simulink subsystem "reference_generator"  (R2020a)
settings: Solver=VariableStepAuto  StartTime=0.0  StopTime=10.0  RelTol=1e-3
model mask{x_params=0, y_params=0, depth_params=0, abs_yaw_params=0, distance=0, desired_lat_vel=0, lat_vel_error_gain=0, counter_max=0}
  mask prompts: x_params "X"; y_params "Y"; depth_params "Depth"; abs_yaw_params "Abs. Yaw"; distance "Distance from pylon"; desired_lat_vel "Desired Lat. Velocity"; lat_vel_error_gain "Lat. Velocity Error Gain"; counter_max "Number of transepts"
undefined symbols (not defined in the file): bool_inspection, misu_Ts, pylonCenter, speed
libraries: simulink x1
settings Model: Creator=andrea  LastModifiedBy=stefano

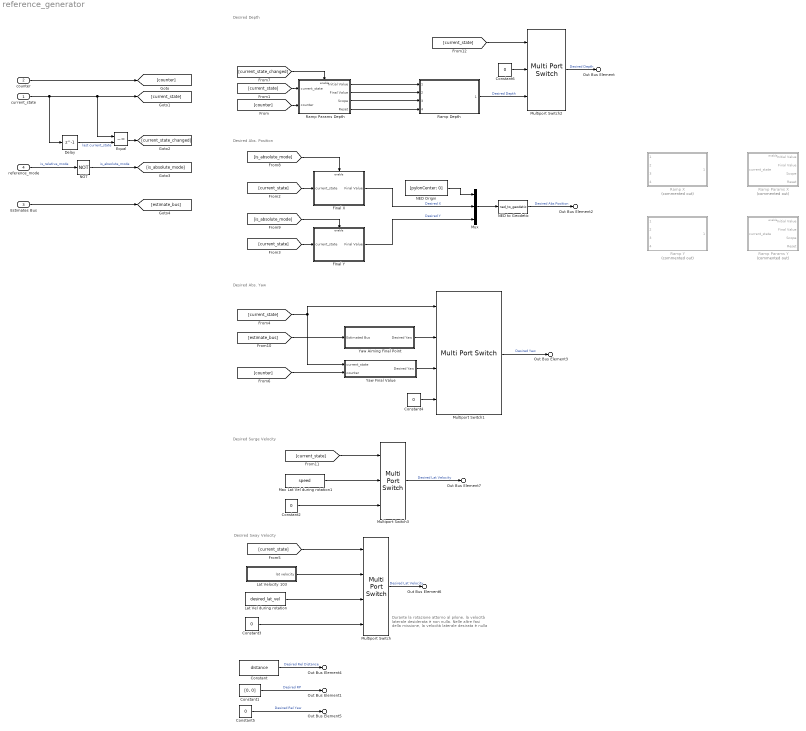
== system reference_generator ==
  note: Desired Surge Velocity
  note: Desired Abs. Yaw
  note: Desired Abs. Position
  note: Desired Depth
  note: Desired Sway Velocity
  note: Durante la rotazione attorno al pilone, la velocità laterale desiderata
      | è non nulla. Nelle altre fasi della missione, la velocità laterale desirata è nulla
  current_state : Inport
  counter : Inport  Port=2
  "Estimates Bus " : Inport  Port=3
  reference_mode : Inport  Port=4
  Constant : Constant  Value=distance
  Constant1 : Constant  Value=[0, 0]
  Constant{2..6} (5 alike) : Constant  Value=0
  Delay : Delay  DelayLength=1
  Equal : RelationalOperator  Operator=~=  OutDataTypeStr=boolean  RndMeth=Simplest
  FInal Y : Subsystem
  Final X : Subsystem
  Lat Vel during rotation : Constant  Value=desired_lat_vel
  Lat Velocity 103 : Subsystem
  Max Lat Vel during rotation1 : Constant  Value=speed
  Multiport Switch : MultiPortSwitch  DataPortOrder=Specify indices  DataPortIndices={103, 202, 201}  DiagnosticForDefault=None
  Multiport Switch1 : MultiPortSwitch  DataPortOrder=Specify indices  DataPortIndices={102, [101, 103, 104, 201, 202, 401]}  DataPortForDefault=Additional data port  DiagnosticForDefault=None
  Multiport Switch2 : MultiPortSwitch  DataPortOrder=Specify indices  DataPortIndices={500, 0}  DiagnosticForDefault=None
  Multiport Switch3 : MultiPortSwitch  DataPortOrder=Specify indices  DataPortIndices={[102], 201}  DiagnosticForDefault=None
  Mux : Mux  Inputs=3
  NED Origin : Constant  Value=[pylonCenter; 0]
  NED to Geodetic : MATLABFcn  MATLABFcn=ned_to_geodetic
  NOT : Logic  Operator=NOT  AllPortsSameDT=off  OutDataTypeStr=boolean
  Ramp Depth : Subsystem  ReferencedSubsystem=ramp_generator
  Ramp Params Depth : Subsystem
  Ramp Params X : Subsystem  Commented=on
  Ramp Params Y : Subsystem  Commented=on
  Ramp X : Subsystem  Commented=on  ReferencedSubsystem=ramp_generator
  Ramp Y : Subsystem  Commented=on  ReferencedSubsystem=ramp_generator
  Yaw Aiming Final Point : Subsystem
  Yaw Final Value : Subsystem
  Out Bus Element : Outport  PortName=Desired  Element=Depth
  Out Bus Element1 : Outport  PortName=Desired  Element=RollPitch
  Out Bus Element2 : Outport  PortName=Desired  Element=Abs Position
  Out Bus Element3 : Outport  PortName=Desired  Element=Yaw
  Out Bus Element4 : Outport  PortName=Desired  Element=Rel Distance
  Out Bus Element5 : Outport  PortName=Desired  Element=Rel Orientation
  Out Bus Element6 : Outport  PortName=Desired  Element=Sway Velocity
  Out Bus Element7 : Outport  PortName=Desired  Element=Surge Velocity
  wires:
  "Estimates Bus "/1 -> [estimate_bus]
  Ramp Params Depth/1(Initial Value) -> Ramp Depth/1
  Ramp Params Depth/4(Reset) -> Ramp Depth/4
  FInal Y/1(Final Value) -> Mux/3  "Desired Y"
  Constant/1 -> Out Bus Element4/1  "Desired Rel Distance"
  Constant5/1 -> Out Bus Element5/1  "Desired Rel Yaw"
  Final X/1(Final Value) -> Mux/2  "Desired X"
  Mux/1 -> NED to Geodetic/1
  Ramp Params Depth/3(Scope) -> Ramp Depth/3
  Ramp Depth/1 -> Multiport Switch2/3  "Desired Depth"
  Multiport Switch1/1 -> Out Bus Element3/1  "Desired Yaw"
  Constant1/1 -> Out Bus Element1/1  "Desired RP"
  Ramp Params Depth/2(Final Value) -> Ramp Depth/2
  current_state/1 -> Delay/1, [current_state], Equal/1
  counter/1 -> [counter]
  NED to Geodetic/1 -> Out Bus Element2/1  "Desired Abs Position"
  NED Origin/1 -> Mux/1
  [counter] -> Ramp Params Depth/2(counter)
  [current_state] -> Ramp Params Depth/1(current_state)
  [current_state] -> Final X/1(current_state)
  [current_state] -> FInal Y/1(current_state)
  [current_state] -> Multiport Switch1/1, Yaw Final Value/1(current_state)
  [counter] -> Yaw Final Value/2(counter)
  Delay/1 -> Equal/2  "last current_state"
  Equal/1 -> [current_state_changed]
  [current_state_changed] -> Ramp Params Depth/Enable
  reference_mode/1 -> NOT/1  "is_relative_mode"
  [is_absolute_mode] -> Final X/Enable
  NOT/1 -> [is_absolute_mode]  "is_absolute_mode"
  Multiport Switch/1 -> Out Bus Element6/1  "Desired Lat Velocity"
  [current_state] -> Multiport Switch/1
  Lat Vel during rotation/1 -> Multiport Switch/3
  Constant3/1 -> Multiport Switch/4
  Yaw Aiming Final Point/1(Desired Yaw) -> Multiport Switch1/2
  Yaw Final Value/1(Desired Yaw) -> Multiport Switch1/3
  Constant4/1 -> Multiport Switch1/4
  [estimate_bus] -> Yaw Aiming Final Point/1(Estimated Bus)
  [is_absolute_mode] -> FInal Y/Enable
  [current_state] -> Multiport Switch2/1
  Multiport Switch2/1 -> Out Bus Element/1  "Desired Depth"
  Constant6/1 -> Multiport Switch2/2
  Multiport Switch3/1 -> Out Bus Element7/1  "Desired Lat Velocity"
  Max Lat Vel during rotation1/1 -> Multiport Switch3/2
  Constant2/1 -> Multiport Switch3/3
  [current_state] -> Multiport Switch3/1
  Lat Velocity 103/1(lat velocity) -> Multiport Switch/2

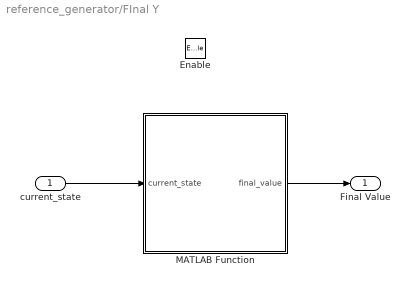
== system reference_generator/FInal Y ==
  current_state : Inport
  Enable : EnablePort
  MATLAB Function : MATLAB Function  TreatAsAtomicUnit=on
  Final Value : Outport
  wires:
  current_state/1 -> MATLAB Function/1(current_state)
  MATLAB Function/1(final_value) -> Final Value/1

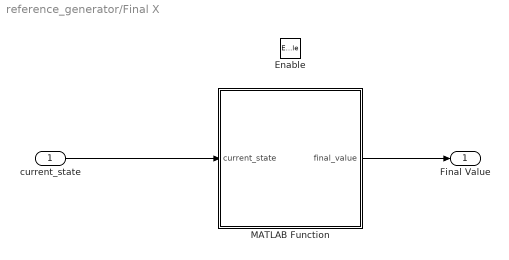
== system reference_generator/Final X ==
  current_state : Inport
  Enable : EnablePort
  MATLAB Function : MATLAB Function  TreatAsAtomicUnit=on
  Final Value : Outport
  wires:
  current_state/1 -> MATLAB Function/1(current_state)
  MATLAB Function/1(final_value) -> Final Value/1

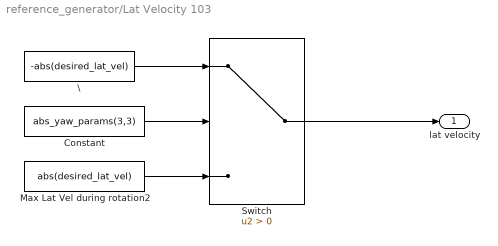
== system reference_generator/Lat Velocity 103 ==
  Constant : Constant  Value=abs_yaw_params(3,3)
  Max Lat Vel during rotation2 : Constant  Value=abs(desired_lat_vel)
  Switch : Switch  Criteria=u2 > Threshold
  \ : Constant  Value=-abs(desired_lat_vel)
  lat velocity : Outport
  wires:
  Switch/1 -> lat velocity/1
  \/1 -> Switch/1
  Max Lat Vel during rotation2/1 -> Switch/3
  Constant/1 -> Switch/2

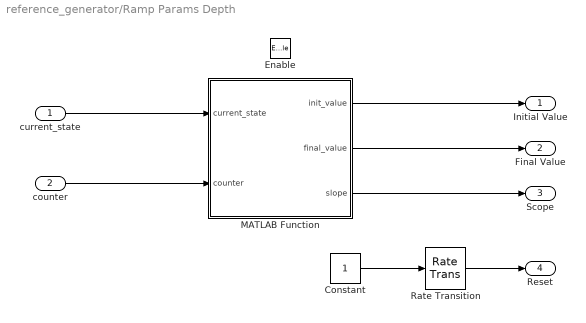
== system reference_generator/Ramp Params Depth ==
  current_state : Inport
  counter : Inport  Port=2
  Enable : EnablePort
  Constant : Constant
  MATLAB Function : MATLAB Function  TreatAsAtomicUnit=on
  Rate Transition : RateTransition  OutPortSampleTime=misu_Ts
  Initial Value : Outport
  Final Value : Outport  Port=2
  Scope : Outport  Port=3
  Reset : Outport  Port=4  OutputWhenDisabled=reset  InitialOutput=0
  wires:
  Rate Transition/1 -> Reset/1
  MATLAB Function/3(slope) -> Scope/1
  MATLAB Function/2(final_value) -> Final Value/1
  MATLAB Function/1(init_value) -> Initial Value/1
  Constant/1 -> Rate Transition/1
  counter/1 -> MATLAB Function/2(counter)
  current_state/1 -> MATLAB Function/1(current_state)

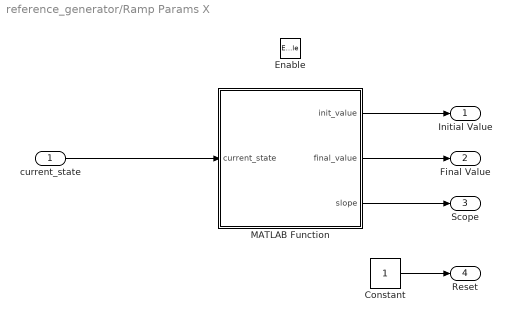
== system reference_generator/Ramp Params X ==
  current_state : Inport
  Enable : EnablePort
  Constant : Constant
  MATLAB Function : MATLAB Function  TreatAsAtomicUnit=on
  Initial Value : Outport
  Final Value : Outport  Port=2
  Scope : Outport  Port=3
  Reset : Outport  Port=4  OutputWhenDisabled=reset  InitialOutput=0
  wires:
  current_state/1 -> MATLAB Function/1(current_state)
  Constant/1 -> Reset/1
  MATLAB Function/3(slope) -> Scope/1
  MATLAB Function/2(final_value) -> Final Value/1
  MATLAB Function/1(init_value) -> Initial Value/1

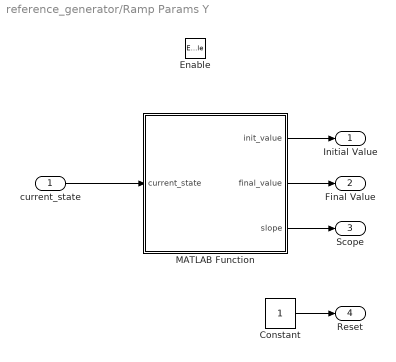
== system reference_generator/Ramp Params Y ==
  current_state : Inport
  Enable : EnablePort
  Constant : Constant
  MATLAB Function : MATLAB Function  TreatAsAtomicUnit=on
  Initial Value : Outport
  Final Value : Outport  Port=2
  Scope : Outport  Port=3
  Reset : Outport  Port=4  OutputWhenDisabled=reset  InitialOutput=0
  wires:
  current_state/1 -> MATLAB Function/1(current_state)
  Constant/1 -> Reset/1
  MATLAB Function/3(slope) -> Scope/1
  MATLAB Function/2(final_value) -> Final Value/1
  MATLAB Function/1(init_value) -> Initial Value/1

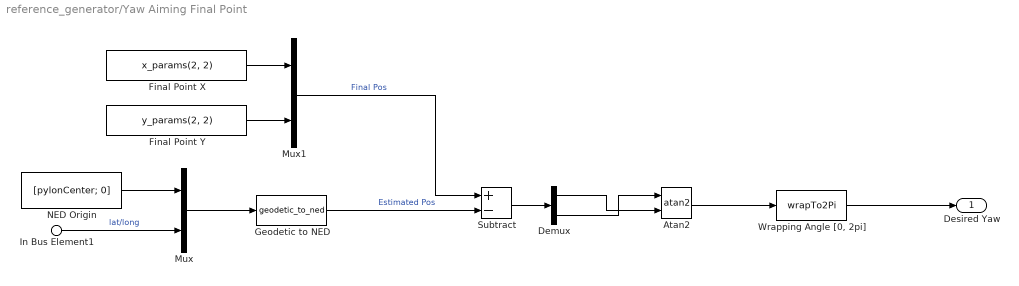
== system reference_generator/Yaw Aiming Final Point ==
  In Bus Element1 : Inport  PortName=Estimated Bus  Element=Estimated Abs Position
  Atan2 : Trigonometry  Operator=atan2
  Demux : Demux  Outputs=2
  Final Point X : Constant  Value=x_params(2, 2)
  Final Point Y : Constant  Value=y_params(2, 2)
  Geodetic to NED : MATLABFcn  MATLABFcn=geodetic_to_ned
  Mux : Mux  Inputs=2
  Mux1 : Mux  Inputs=2
  NED Origin : Constant  Value=[pylonCenter; 0]
  Subtract : Sum  Inputs=+-
  "Wrapping Angle [0, 2pi]" : MATLABFcn  MATLABFcn=wrapTo2Pi  OutputDimensions=1
  Desired Yaw : Outport
  wires:
  "Wrapping Angle [0, 2pi]"/1 -> Desired Yaw/1
  Atan2/1 -> "Wrapping Angle [0, 2pi]"/1
  Subtract/1 -> Demux/1
  Mux1/1 -> Subtract/1  "Final Pos"
  Final Point Y/1 -> Mux1/2
  Final Point X/1 -> Mux1/1
  Geodetic to NED/1 -> Subtract/2  "Estimated Pos"
  In Bus Element1/1 -> Mux/2  "lat/long"
  Mux/1 -> Geodetic to NED/1
  NED Origin/1 -> Mux/1
  Demux/1 -> Atan2/2
  Demux/2 -> Atan2/1

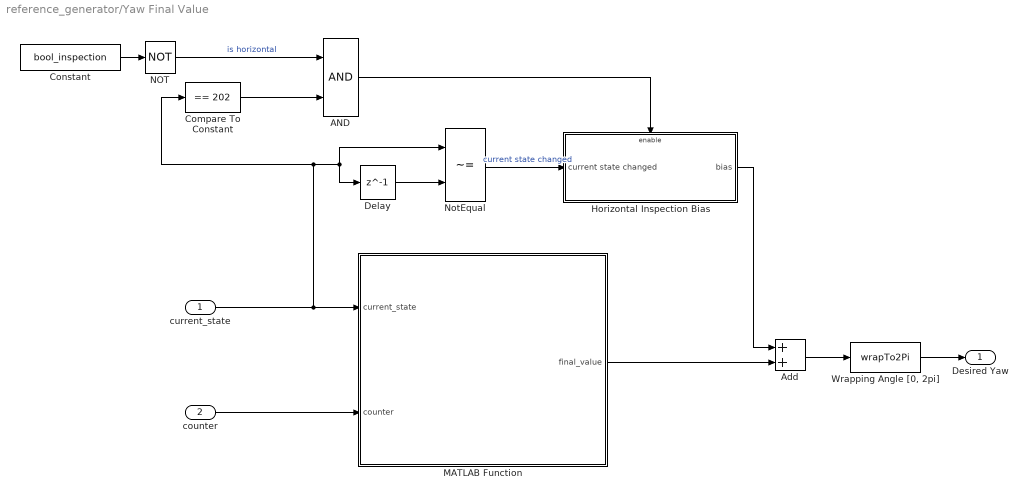
== system reference_generator/Yaw Final Value ==
  current_state : Inport
  counter : Inport  Port=2
  AND : Logic  IconShape=distinctive  AllPortsSameDT=off  OutDataTypeStr=boolean
  Add : Sum
  Compare To Constant : simulink/Logic and Bit Operations/Compare To Constant  relop===  const=202  OutDataTypeStr=boolean
  Constant : Constant  Value=bool_inspection
  Delay : Delay  DelayLength=1
  Horizontal Inspection Bias : Subsystem
  MATLAB Function : MATLAB Function  TreatAsAtomicUnit=on
  NOT : Logic  Operator=NOT  IconShape=distinctive  AllPortsSameDT=off  OutDataTypeStr=boolean
  NotEqual : RelationalOperator  Operator=~=  OutDataTypeStr=boolean  RndMeth=Simplest
  "Wrapping Angle [0, 2pi]" : MATLABFcn  MATLABFcn=wrapTo2Pi
  Desired Yaw : Outport
  wires:
  NotEqual/1 -> Horizontal Inspection Bias/1(current state changed)  "current state changed"
  Delay/1 -> NotEqual/2
  current_state/1 -> MATLAB Function/1(current_state), Delay/1, NotEqual/1, Compare To Constant/1
  AND/1 -> Horizontal Inspection Bias/Enable
  Compare To Constant/1 -> AND/2
  NOT/1 -> AND/1  "is horizontal"
  Constant/1 -> NOT/1
  Horizontal Inspection Bias/1(bias) -> Add/1
  "Wrapping Angle [0, 2pi]"/1 -> Desired Yaw/1
  Add/1 -> "Wrapping Angle [0, 2pi]"/1
  MATLAB Function/1(final_value) -> Add/2
  counter/1 -> MATLAB Function/2(counter)

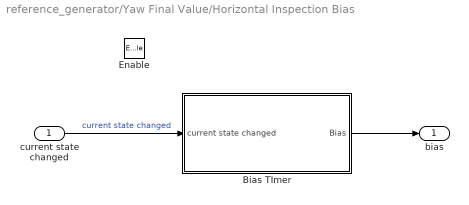
== system reference_generator/Yaw Final Value/Horizontal Inspection Bias ==
  current state changed : Inport
  Enable : EnablePort
  Bias TImer : Subsystem
  bias : Outport  OutputWhenDisabled=reset  InitialOutput=0
  wires:
  Bias TImer/1(Bias) -> bias/1
  current state changed/1 -> Bias TImer/1(current state changed)  "current state changed"

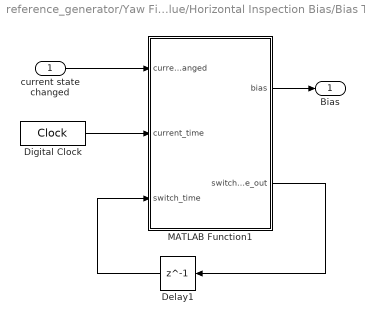
== system reference_generator/Yaw Final Value/Horizontal Inspection Bias/Bias TImer ==
  current state changed : Inport
  Delay1 : Delay  DelayLength=1
  Digital Clock : DigitalClock  SampleTime=misu_Ts
  MATLAB Function1 : MATLAB Function  TreatAsAtomicUnit=on
  Bias : Outport
  wires:
  current state changed/1 -> MATLAB Function1/1(current_state_changed)
  MATLAB Function1/2(switch_time_out) -> Delay1/1
  MATLAB Function1/1(bias) -> Bias/1
  Digital Clock/1 -> MATLAB Function1/2(current_time)
  Delay1/1 -> MATLAB Function1/3(switch_time)

== matlab function reference_generator/FInal Y/MATLAB Function ==
  data: current_state input; final_value output; y_params parameter
function final_value  = y_params_lookup(current_state, y_params)

row_index = checkpoint_row_index(current_state, 0, 0);
if row_index ~= -1
    final_value = y_params(row_index, 2);
else
    final_value = 0;
end

end

== matlab function reference_generator/Final X/MATLAB Function ==
  data: current_state input; final_value output; x_params parameter
function final_value  = x_params_lookup(current_state, x_params)

row_index = checkpoint_row_index(current_state, 0, 0);
if row_index ~= -1
    final_value = x_params(row_index, 2);
else
    final_value = 0;
end

end

== matlab function reference_generator/Ramp Params Depth/MATLAB Function ==
  data: current_state input; init_value output; counter input; depth_params parameter; counter_max parameter; final_value output; slope output
function [init_value, final_value, slope] = depth_params_lookup(current_state, counter, depth_params, counter_max)

row_index = checkpoint_row_index(current_state, counter, counter_max);
if row_index ~= -1
    init_value = depth_params(row_index, 1);
    final_value = depth_params(row_index, 2);
    slope = depth_params(row_index, 3);
else
    init_value = 0;
    final_value = 0;
    slope = 0;
end

end

== matlab function reference_generator/Ramp Params X/MATLAB Function ==
  data: current_state input; init_value output; final_value output; slope output; x_params parameter
function [init_value, final_value, slope] = x_params_lookup(current_state, x_params)

row_index = checkpoint_row_index(current_state, 0, 0);
if row_index ~= -1
    init_value = x_params(row_index, 1);
    final_value = x_params(row_index, 2);
    slope = x_params(row_index, 3);
else
    init_value = 0;
    final_value = 0;
    slope = 0;
end

end

== matlab function reference_generator/Ramp Params Y/MATLAB Function ==
  data: current_state input; init_value output; final_value output; slope output; y_params parameter
function [init_value, final_value, slope] = y_params_lookup(current_state, y_params)

row_index = checkpoint_row_index(current_state, 0, 0);
if row_index ~= -1
    init_value = y_params(row_index, 1);
    final_value = y_params(row_index, 2);
    slope = y_params(row_index, 3);
else
    init_value = 0;
    final_value = 0;
    slope = 0;
end

end

== matlab function reference_generator/Yaw Final Value/Horizontal Inspection Bias/Bias TImer/MATLAB Function1 ==
  data: bias output; switch_time_out output; current_state_changed input; current_time input; switch_time input
function [bias, switch_time_out]= fcn(current_state_changed, current_time, switch_time)

if current_state_changed
    switch_time = current_time + 20;
end
switch_time_out = switch_time;

if current_time >= switch_time
    bias = 0;
else
    bias = pi;
end

== matlab function reference_generator/Yaw Final Value/MATLAB Function ==
  data: current_state input; final_value output size=1; counter_max parameter; counter input; abs_yaw_params parameter
function final_value = abs_yaw_final_value_lookup(current_state, counter_max, counter, abs_yaw_params)

row_index = checkpoint_row_index(current_state, counter, counter_max);

if row_index ~= -1
    final_value = abs_yaw_params(row_index, 2);
else
    final_value = 0;
end

end
